simulink model "sf_call_c"  (R2021a)
settings: Solver=FixedStepDiscrete  StartTime=0.0  StopTime=10.0  RelTol=1e-3
PreLoadFcn:
  | Simulink.importExternalCTypes('ex_myTypes_LCT.h');
  | param = struct;
  | param.param1 = 15;
  | param.param2 = 15;
  | param.param3 = 15;
CloseFcn:
  | try
  | rmdir slprj\ s
  | catch
  | end
  | try
  | folder_name = [bdroot '*'];
  | rmdir(folder_name,'s')
  | catch
  | end
  | try
  | file_temp_name = [bdroot '.slxc'];
  | delete(file_temp_name)
  | catch
  | end
  | clear folder_name file_temp_name
settings Model: Creator=jetson  LastModifiedBy=jetson
settings DataIOCC: SaveOutput=off  SignalLogging=off  DSMLogging=off  SaveTime=off  ReturnWorkspaceOutputs=off
settings OptimizationCC: DefaultParameterBehavior=Inlined  EnhancedBackFolding=on  PassReuseOutputArgsAs=Individual arguments  ZeroExternalMemoryAtStartup=off  ZeroInternalMemoryAtStartup=off  OptimizeBlockOrder=speed  DifferentSizesBufferReuse=on  OptimizationCustomize=off  EfficientTunableParamExpr=on
settings DebuggingCC: ParameterTunabilityLossMsg=error
settings SFSimCC: SimCustomHeaderCode="#include\"ex_myTypes_LCT.h\""  SimUserSources=ex_mySrc_LCT.c  MATLABDynamicMemAlloc=off
settings RTWCC: SystemTargetFile=ert.tlc  GenCodeOnly=on  TemplateMakefile=ert_default_tmf  GenerateReport=on  RTWUseSimCustomCode=on  CustomHeaderCode="#include\"ex_myTypes_LCT.h\""  CustomSource=ex_mySrc_LCT.c  IncludeHyperlinkInReport=on  LaunchReport=on  GenerateTraceInfo=on
settings CodeAppCC: ForceParamTrailComments=on  IgnoreCustomStorageClasses=off  OperatorAnnotations=on  SimulinkDataObjDesc=on  SFDataObjDesc=on  InsertBlockDesc=on
settings ERTTargetCC: TargetLangStandard=C99 (ISO)  GenerateSampleERTMain=on  InlinedParameterPlacement=NonHierarchical  ERTCustomFileTemplate=example_file_process.tlc

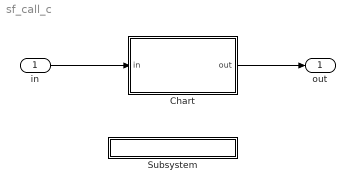
== system sf_call_c ==
  in : Inport  ClipboardFcn=Data Type : %<OutDataTypeStr>  OutDataTypeStr=Bus: sigStructType
      settings: AttributesFormatString=Data Type : %<OutDataTypeStr>
  Chart : Stateflow chart  TreatAsAtomicUnit=on
  Subsystem : Subsystem
      settings: OpenFcn=web(fullfile(docroot, 'simulink/sfg/integrating-existing-c-functions-into-simulink-models-with-the-legacy-code-tool.html'))
      mask Display: disp('double click open help')
  out : Outport  OutDataTypeStr=Bus: sigStructType
      settings: AttributesFormatString=Data Type : %<OutDataTypeStr>
  wires:
  in/1 -> Chart/1(in)
  Chart/1(out) -> out/1

== system sf_call_c/Subsystem ==

== stateflow chart sf_call_c/Chart ==
  (default) -> (junction 4) : {myFcn(&in,&param,&out);}
  data: in input Bus: sigStructType size=1; out output Bus: sigStructType size=1; param parameter Bus: paramStructType size=1
